simulink model "MF_simula_disc_teste"  (R2012b)
settings: Solver=ode3  StartTime=0  StopTime=Tsim  FixedStep=1e-7  RelTol=1e-3
values from neighbouring files (symbols this model uses):
  D0 = 0.3    [MA_roda_sim.m]    (also in MF_roda_sim_disc.m; sim_padrao.mat = [0.344368016885 0.340474742468 0.337081858539 0.333995318743)
  dc = [1 0]    [MF_roda_sim_disc.m]
  dD = 0.0    (= 0)    [MA_roda_sim.m]
  dref = 10    [MF_roda_sim_disc.m]
  dVin = 2    [MA_roda_sim.m]    (also in MF_roda_sim_disc.m)
  nc = [0.000087830589033 3.757361353061334]    [MF_roda_sim_disc.m]
  ref = 90    [MF_roda_sim_disc.m]
  Ta = 1/fa    (= 1e-05)    [MF_roda_sim_disc.m]
  tdD = Tsim/3    (= 0.0333333333333)    [MA_roda_sim.m]
  tdVin = 2*Tsim/3    (= 0.0666666666667)    [MA_roda_sim.m]    (also in MF_roda_sim_disc.m = 0.2)
  tref = Tsim/3    (= 0.1)    [MF_roda_sim_disc.m]
  Vin0 = 15.5    [MA_roda_sim.m]    (also in MF_roda_sim_disc.m)
undefined symbols (not defined in the file or in its folder): A_linear, B_mimo, C, dd, nd, xss
settings Model: CovModelRefEnable=off  Creator=jv_flores  LastModifiedBy=anton
settings DataIOCC: LimitDataPoints=off  SaveFormat=StructureWithTime
settings OptimizationCC: ExpressionDepthLimit=128
settings DebuggingCC: UnderspecifiedInitializationDetection=Simplified  MergeDetectMultiDrivingBlocksExec=error  SolverPrmCheckMsg=none  FrameProcessingCompatibilityMsg=error  StateNameClashWarn=none
settings HardwareCC: ProdBitPerPointer=64  ProdLargestAtomicFloat=Float  ProdIntDivRoundTo=Zero  ProdEndianess=LittleEndian  ProdHWDeviceType=Specified
settings ModelReferenceCC: PropagateSignalLabelsOutOfModel=on
settings CodeAppCC: CustomSymbolStrType=$N$R$M_T
settings GRTTargetCC: CodeReplacementLibrary=C89/C90 (ANSI)

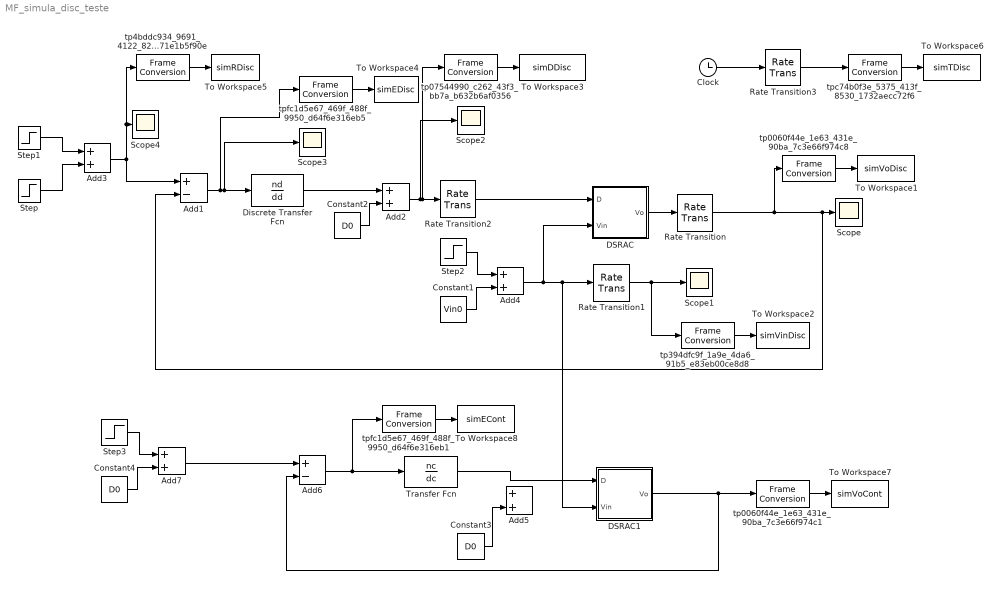
== system MF_simula_disc_teste ==
  Add1 : Sum  Inputs=+-
  Add{2..5,7} (5 alike) : Sum
  Add6 : Sum  Inputs=+-
  Clock : Clock
  Constant1 : Constant  Value=Vin0
  Constant2 : Constant  Value=D0  SampleTime=Ta
  Constant3 : Constant  Value=D0  SampleTime=Ta
  Constant4 : Constant  Value=D0
  DSRAC : Subsystem
  DSRAC1 : Subsystem
  Discrete Transfer Fcn : DiscreteTransferFcn  Numerator=nd  Denominator=dd  SampleTime=Ta
  Rate Transition : RateTransition  OutPortSampleTime=Ta
  Rate Transition1 : RateTransition  OutPortSampleTime=Ta
  Rate Transition2 : RateTransition  OutPortSampleTimeOpt=Inherit
  Rate Transition3 : RateTransition  OutPortSampleTime=Ta
  Scope{,1..4} (5 alike) : Scope
      Scope settings: YMin=84.67462  YMax=121.55969  SaveName=simVoDisc  SampleInput=on  SampleTime=Ta
      Scope1 settings: YMin=15.25  YMax=17.75  SaveName=simVinDisc
      Scope2 settings: YMin=0.14485  YMax=0.58464  SaveName=simDDisc  SampleInput=on  SampleTime=Ta
      Scope3 settings: YMin=-20.93469  YMax=9.70038  SaveName=simEDisc  SampleInput=on  SampleTime=Ta
      Scope4 settings: YMin=0.14485  YMax=0.58464  SaveName=simRDisc  SampleInput=on  SampleTime=Ta
  Step : Step  Time=0  After=ref  SampleTime=Ta
  Step1 : Step  Time=tref  After=dref  SampleTime=Ta
  Step2 : Step  Time=tdVin  After=dVin  SampleTime=0
  Step3 : Step  Time=tdD  After=dD  SampleTime=0
  To Workspace1 : ToWorkspace  VariableName=simVoDisc  SampleTime=Ta
  To Workspace2 : ToWorkspace  VariableName=simVinDisc  SampleTime=Ta
  To Workspace3 : ToWorkspace  VariableName=simDDisc  SampleTime=Ta
  To Workspace4 : ToWorkspace  VariableName=simEDisc  SampleTime=Ta
  To Workspace5 : ToWorkspace  VariableName=simRDisc  SampleTime=Ta
  To Workspace6 : ToWorkspace  VariableName=simTDisc  SampleTime=Ta
  To Workspace7 : ToWorkspace  VariableName=simVoCont  SampleTime=Ta
  To Workspace8 : ToWorkspace  VariableName=simECont  SampleTime=Ta
  Transfer Fcn : TransferFcn  Numerator=nc  Denominator=dc
  tp0060f44e_1e63_431e_90ba_7c3e66f974c1 : FrameConversion  OutFrame=Sample-based
  tp0060f44e_1e63_431e_90ba_7c3e66f974c8 : FrameConversion  OutFrame=Sample-based
  tp07544990_c262_43f3_bb7a_b632b6af0356 : FrameConversion  OutFrame=Sample-based
  tp394dfc9f_1a9e_4da6_91b5_e83eb00ce8d8 : FrameConversion  OutFrame=Sample-based
  tp4bddc934_9691_4122_82e3_0371e1b5f90e : FrameConversion  OutFrame=Sample-based
  tpc74b0f3e_5375_413f_8530_1732aecc72f6 : FrameConversion  OutFrame=Sample-based
  tpfc1d5e67_469f_488f_9950_d64f6e316eb1 : FrameConversion  OutFrame=Sample-based
  tpfc1d5e67_469f_488f_9950_d64f6e316eb5 : FrameConversion  OutFrame=Sample-based
  wires:
  DSRAC/1(Vo) -> Rate Transition/1
  Constant2/1 -> Add2/2
  Rate Transition/1 -> Add1/2, Scope/1, tp0060f44e_1e63_431e_90ba_7c3e66f974c8/1
  Rate Transition1/1 -> Scope1/1, tp394dfc9f_1a9e_4da6_91b5_e83eb00ce8d8/1
  Add1/1 -> Discrete Transfer Fcn/1, Scope3/1, tpfc1d5e67_469f_488f_9950_d64f6e316eb5/1
  Rate Transition2/1 -> DSRAC/1(D)
  Discrete Transfer Fcn/1 -> Add2/1
  Step1/1 -> Add3/1
  Step/1 -> Add3/2
  Add3/1 -> tp4bddc934_9691_4122_82e3_0371e1b5f90e/1, Scope4/1, Add1/1
  Add2/1 -> tp07544990_c262_43f3_bb7a_b632b6af0356/1, Rate Transition2/1, Scope2/1
  Clock/1 -> Rate Transition3/1
  Step2/1 -> Add4/1
  Constant1/1 -> Add4/2
  Add4/1 -> DSRAC/2(Vin), DSRAC1/2(Vin), Rate Transition1/1
  tp0060f44e_1e63_431e_90ba_7c3e66f974c8/1 -> To Workspace1/1
  tp394dfc9f_1a9e_4da6_91b5_e83eb00ce8d8/1 -> To Workspace2/1
  tp07544990_c262_43f3_bb7a_b632b6af0356/1 -> To Workspace3/1
  tpfc1d5e67_469f_488f_9950_d64f6e316eb5/1 -> To Workspace4/1
  tp4bddc934_9691_4122_82e3_0371e1b5f90e/1 -> To Workspace5/1
  Rate Transition3/1 -> tpc74b0f3e_5375_413f_8530_1732aecc72f6/1
  tpc74b0f3e_5375_413f_8530_1732aecc72f6/1 -> To Workspace6/1
  Constant3/1 -> Add5/2
  tp0060f44e_1e63_431e_90ba_7c3e66f974c1/1 -> To Workspace7/1
  DSRAC1/1(Vo) -> tp0060f44e_1e63_431e_90ba_7c3e66f974c1/1, Add6/2
  Add6/1 -> tpfc1d5e67_469f_488f_9950_d64f6e316eb1/1, Transfer Fcn/1
  tpfc1d5e67_469f_488f_9950_d64f6e316eb1/1 -> To Workspace8/1
  Transfer Fcn/1 -> DSRAC1/1(D)
  Step3/1 -> Add7/1
  Constant4/1 -> Add7/2
  Add7/1 -> Add6/1

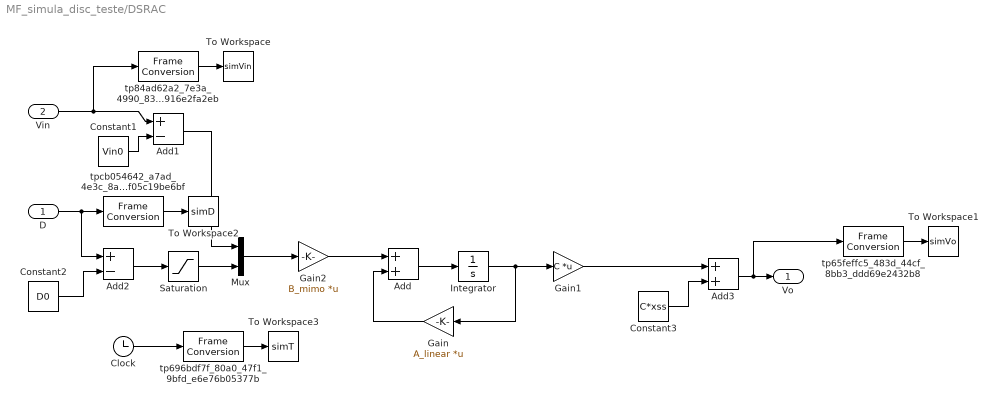
== system MF_simula_disc_teste/DSRAC ==
  D : Inport
  Vin : Inport  Port=2
  Add : Sum
  Add1 : Sum  Inputs=+-
  Add2 : Sum  Inputs=+-
  Add3 : Sum
  Clock : Clock
  Constant1 : Constant  Value=Vin0
  Constant2 : Constant  Value=D0
  Constant3 : Constant  Value=C*xss
  Gain : Gain  Gain=A_linear  Multiplication=Matrix(K*u)
  Gain1 : Gain  Gain=C  Multiplication=Matrix(K*u)
  Gain2 : Gain  Gain=B_mimo  Multiplication=Matrix(K*u)
  Integrator : Integrator
  Mux : Mux  Inputs=2
  Saturation : Saturate  UpperLimit=1  LowerLimit=0
  To Workspace : ToWorkspace  VariableName=simVin  SampleTime=-1
  To Workspace1 : ToWorkspace  VariableName=simVo  SampleTime=-1
  To Workspace2 : ToWorkspace  VariableName=simD  SampleTime=-1
  To Workspace3 : ToWorkspace  VariableName=simT  SampleTime=-1
  tp65feffc5_483d_44cf_8bb3_ddd69e2432b8 : FrameConversion  OutFrame=Sample-based
  tp696bdf7f_80a0_47f1_9bfd_e6e76b05377b : FrameConversion  OutFrame=Sample-based
  tp84ad62a2_7e3a_4990_8314_19916e2fa2eb : FrameConversion  OutFrame=Sample-based
  tpcb054642_a7ad_4e3c_8a21_0f05c19be6bf : FrameConversion  OutFrame=Sample-based
  Vo : Outport
  wires:
  Gain2/1 -> Add/1
  Add2/1 -> Saturation/1
  Constant2/1 -> Add2/2
  Integrator/1 -> Gain/1, Gain1/1
  Mux/1 -> Gain2/1
  Gain/1 -> Add/2
  Add/1 -> Integrator/1
  Add3/1 -> Vo/1, tp65feffc5_483d_44cf_8bb3_ddd69e2432b8/1
  Gain1/1 -> Add3/1
  Constant3/1 -> Add3/2
  D/1 -> Add2/1, tpcb054642_a7ad_4e3c_8a21_0f05c19be6bf/1
  Saturation/1 -> Mux/2
  Vin/1 -> Add1/1, tp84ad62a2_7e3a_4990_8314_19916e2fa2eb/1
  Constant1/1 -> Add1/2
  Add1/1 -> Mux/1
  tp84ad62a2_7e3a_4990_8314_19916e2fa2eb/1 -> To Workspace/1
  tp65feffc5_483d_44cf_8bb3_ddd69e2432b8/1 -> To Workspace1/1
  tpcb054642_a7ad_4e3c_8a21_0f05c19be6bf/1 -> To Workspace2/1
  Clock/1 -> tp696bdf7f_80a0_47f1_9bfd_e6e76b05377b/1
  tp696bdf7f_80a0_47f1_9bfd_e6e76b05377b/1 -> To Workspace3/1

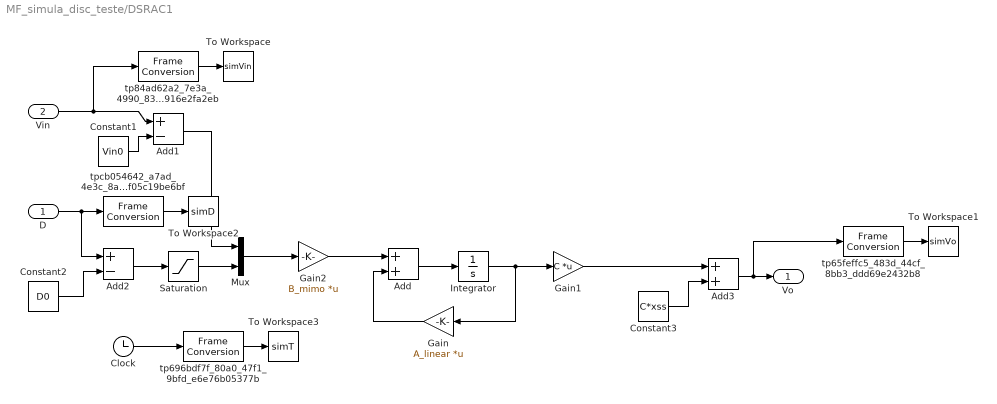
== system MF_simula_disc_teste/DSRAC1 ==
  D : Inport
  Vin : Inport  Port=2
  Add : Sum
  Add1 : Sum  Inputs=+-
  Add2 : Sum  Inputs=+-
  Add3 : Sum
  Clock : Clock
  Constant1 : Constant  Value=Vin0
  Constant2 : Constant  Value=D0
  Constant3 : Constant  Value=C*xss
  Gain : Gain  Gain=A_linear  Multiplication=Matrix(K*u)
  Gain1 : Gain  Gain=C  Multiplication=Matrix(K*u)
  Gain2 : Gain  Gain=B_mimo  Multiplication=Matrix(K*u)
  Integrator : Integrator
  Mux : Mux  Inputs=2
  Saturation : Saturate  UpperLimit=1  LowerLimit=0
  To Workspace : ToWorkspace  VariableName=simVin  SampleTime=-1
  To Workspace1 : ToWorkspace  VariableName=simVo  SampleTime=-1
  To Workspace2 : ToWorkspace  VariableName=simD  SampleTime=-1
  To Workspace3 : ToWorkspace  VariableName=simT  SampleTime=-1
  tp65feffc5_483d_44cf_8bb3_ddd69e2432b8 : FrameConversion  OutFrame=Sample-based
  tp696bdf7f_80a0_47f1_9bfd_e6e76b05377b : FrameConversion  OutFrame=Sample-based
  tp84ad62a2_7e3a_4990_8314_19916e2fa2eb : FrameConversion  OutFrame=Sample-based
  tpcb054642_a7ad_4e3c_8a21_0f05c19be6bf : FrameConversion  OutFrame=Sample-based
  Vo : Outport
  wires:
  Gain2/1 -> Add/1
  Add2/1 -> Saturation/1
  Constant2/1 -> Add2/2
  Integrator/1 -> Gain/1, Gain1/1
  Mux/1 -> Gain2/1
  Gain/1 -> Add/2
  Add/1 -> Integrator/1
  Add3/1 -> Vo/1, tp65feffc5_483d_44cf_8bb3_ddd69e2432b8/1
  Gain1/1 -> Add3/1
  Constant3/1 -> Add3/2
  D/1 -> Add2/1, tpcb054642_a7ad_4e3c_8a21_0f05c19be6bf/1
  Saturation/1 -> Mux/2
  Vin/1 -> Add1/1, tp84ad62a2_7e3a_4990_8314_19916e2fa2eb/1
  Constant1/1 -> Add1/2
  Add1/1 -> Mux/1
  tp84ad62a2_7e3a_4990_8314_19916e2fa2eb/1 -> To Workspace/1
  tp65feffc5_483d_44cf_8bb3_ddd69e2432b8/1 -> To Workspace1/1
  tpcb054642_a7ad_4e3c_8a21_0f05c19be6bf/1 -> To Workspace2/1
  Clock/1 -> tp696bdf7f_80a0_47f1_9bfd_e6e76b05377b/1
  tp696bdf7f_80a0_47f1_9bfd_e6e76b05377b/1 -> To Workspace3/1
